simulink model "system4"  (R2016b)
settings: Solver=FixedStepAuto  StartTime=0.0  StopTime=50  FixedStep=0.0001  RelTol=1e-3
settings Model: Creator=User  LastModifiedBy=akshita_jain

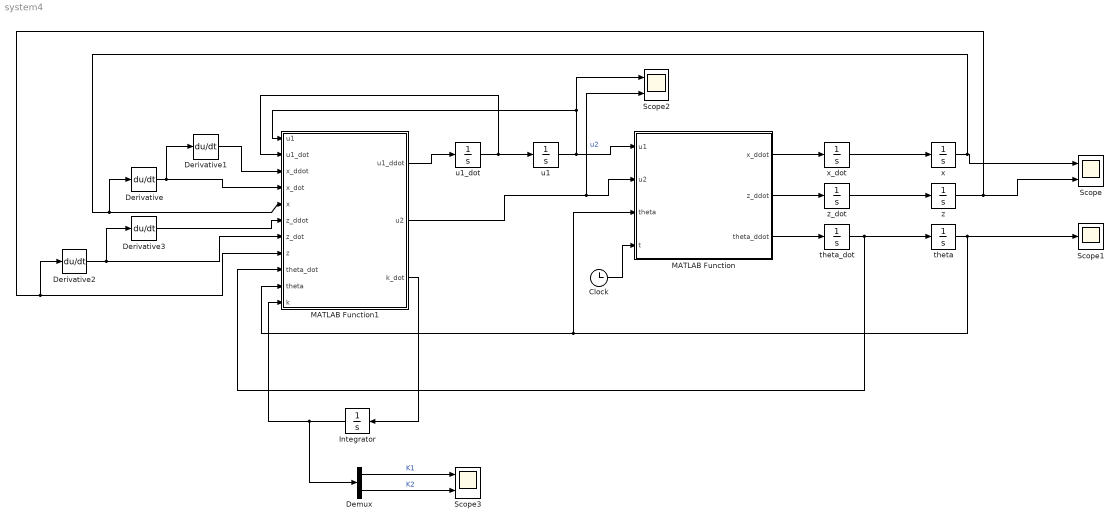
== system system4 ==
  Clock : Clock
      settings: Decimation=100
  Demux : Demux  Outputs=2
  Derivative{,1..3} (4 alike) : Derivative
  Integrator : Integrator  InitialCondition=[1;1]
  MATLAB Function : MATLAB Function  TreatAsAtomicUnit=on
  MATLAB Function1 : MATLAB Function  TreatAsAtomicUnit=on
  Scope : Scope  NumInputPorts=2
  Scope1 : Scope
  Scope2 : Scope  NumInputPorts=2
  Scope3 : Scope  NumInputPorts=2
  theta : Integrator  InitialCondition=pi/4
  theta_dot : Integrator
  u1 : Integrator  InitialCondition=1
  u1_dot : Integrator
  x : Integrator  InitialCondition=2
  x_dot : Integrator
  z : Integrator  InitialCondition=3
  z_dot : Integrator
  wires:
  Derivative3/1 -> MATLAB Function1/6(z_ddot)
  Derivative/1 -> Derivative1/1, MATLAB Function1/4(x_dot)
  MATLAB Function1/1(u1_ddot) -> u1_dot/1
  MATLAB Function/3(theta_ddot) -> theta_dot/1
  x_dot/1 -> x/1
  u1_dot/1 -> MATLAB Function1/2(u1_dot), u1/1
  MATLAB Function/2(z_ddot) -> z_dot/1
  MATLAB Function1/2(u2) -> Scope2/2, MATLAB Function/2(u2)  "u2"
  z_dot/1 -> z/1
  x/1 -> Scope/1, Derivative/1, MATLAB Function1/5(x)
  Derivative2/1 -> Derivative3/1, MATLAB Function1/7(z_dot)
  z/1 -> Scope/2, Derivative2/1, MATLAB Function1/8(z)
  theta_dot/1 -> MATLAB Function1/9(theta_dot), theta/1
  Derivative1/1 -> MATLAB Function1/3(x_ddot)
  Clock/1 -> MATLAB Function/4(t)
  u1/1 -> MATLAB Function1/1(u1), Scope2/1, MATLAB Function/1(u1)
  MATLAB Function/1(x_ddot) -> x_dot/1
  theta/1 -> Scope1/1, MATLAB Function/3(theta), MATLAB Function1/10(theta)
  MATLAB Function1/3(k_dot) -> Integrator/1
  Integrator/1 -> Demux/1, MATLAB Function1/11(k)
  Demux/1 -> Scope3/1  "K1"
  Demux/2 -> Scope3/2  "K2"

== matlab function system4/MATLAB Function1 ==
  data: u1 input; u1_dot input; x_ddot input; x_dot input; u1_ddot output; u2 output; x input; z_ddot input; z_dot input; z input; theta_dot input; theta input; k input; k_dot output
function [u1_ddot, u2, k_dot] = adaptiveSlidingControl(u1, u1_dot, x_ddot, x_dot, x, z_ddot, z_dot, z, theta_dot, theta, k)
%gains
c1 = 3;
c2 = 3;
c3 = 1;

kbar = [300;300];
n = [0.3;0.3];
u = [0.001;0.001];

% state
x_3dot = -u1_dot*sin(theta) - u1*theta_dot*cos(theta);

z_3dot = u1_dot*cos(theta) - u1*theta_dot*sin(theta);

%sliding variable

s = [x_3dot+c1*x_ddot+c2*x_dot+c3*x;
    z_3dot+c1*z_ddot+c2*z_dot+c3*z];

if (k > n)
    k_dot = kbar .* abs(s) .* sign(abs(s)-u);
else
    k_dot = n;
end

beta = [-sin(theta) -u1*cos(theta);
        cos(theta) -u1*sin(theta)];
    
alpha = [-2*u1_dot*cos(theta)*theta_dot+u1*sin(theta)*theta_dot^2+c1*x_3dot+c2*x_ddot+c3*x_dot;
        -2*u1_dot*sin(theta)*theta_dot-u1*cos(theta)*theta_dot^2+c1*z_3dot+c2*z_ddot+c3*z_dot];
    
del = 0.3;
if (abs(s) > del)
    sat = sign(s);
else
    sat = s / del;
end
    
u = beta\(-alpha - k.*sat);
u1_ddot = u(1);
u2 = u(2);

== matlab function system4/MATLAB Function ==
  data: u1 input; x_ddot output; u2 input; z_ddot output; theta_ddot output; theta input; t input
function [x_ddot, z_ddot, theta_ddot] = system(u1,u2,theta, t)

x_ddot = -sin(theta)*u1;
z_ddot = cos(theta)*u1 - 1;
theta_ddot = u2+200*sin(t);
